simulink library "unity_lib_UDP"  (R2021a)
settings: Solver=VariableStepAuto  StartTime=0.0  StopTime=10.0  RelTol=1e-3
libraries: dspnetwork x1
settings Model: Creator=ge26jow  LastModifiedBy=ge26jow

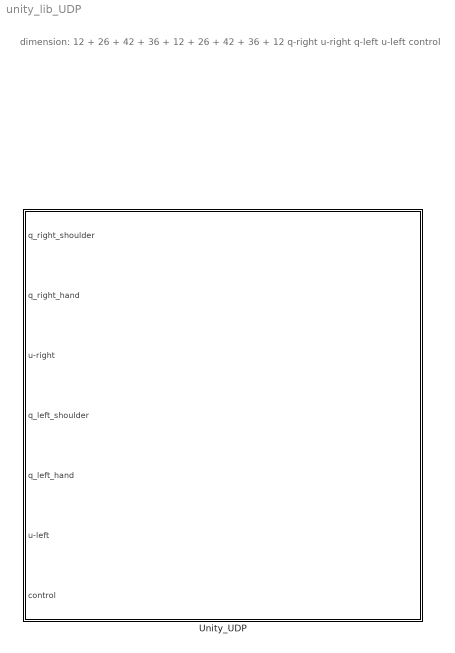
== system unity_lib_UDP ==
  note: dimension:
      |
      | 12 + 26 + 42 + 36 + 12 + 26 + 42 + 36 + 12
      | q-right u-right q-left u-left control
  Unity_UDP : Subsystem  mask{IP_port=8051, sampling_time=1e-2}
      mask prompts: IP_port "IP port"; sampling_time "sampling time"

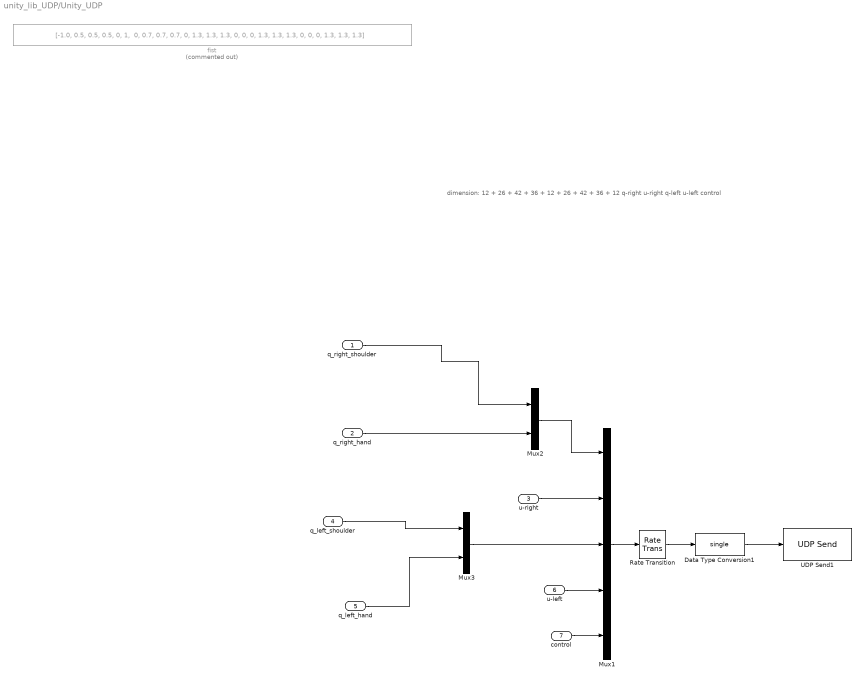
== system unity_lib_UDP/Unity_UDP ==
  note: dimension:
      |
      | 12 + 26 + 42 + 36 + 12 + 26 + 42 + 36 + 12
      | q-right u-right q-left u-left control
  q_right_shoulder : Inport
  q_right_hand : Inport  Port=2
  u-right : Inport  Port=3
  q_left_shoulder : Inport  Port=4
  q_left_hand : Inport  Port=5
  u-left : Inport  Port=6
  control : Inport  Port=7
  Data Type Conversion1 : DataTypeConversion  OutDataTypeStr=single
  Mux1 : Mux  Inputs=[12+26, 42+36, 12+26, 42+36, 12]
  Mux2 : Mux  Inputs=[12, 26]
  Mux3 : Mux  Inputs=[12, 26]
  Rate Transition : RateTransition  OutPortSampleTime=sampling_time
  UDP Send1 : dspnetwork/UDP Send  remoteURL='127.0.0.1'  remotePort=IP_port  localURL='0.0.0.0'  localPortSource=Automatically determine  localPort=-1  sendBufferSize=8192  sampletime=-1  blockPlatform=[]  separateLengthPort=0
      settings: SourceProductBaseCode=DS
  fist : Constant  Commented=on  Value="[-1.0, 0.5, 0.5, 0.5, 0, 1,  0, 0.7, 0.7, 0.7, 0, 1.3, 1.3, 1.3, 0, 0, 0, 1.3, 1.3, 1.3, 0, 0, 0, 1.3, 1.3, 1.3]"
  wires:
  q_right_hand/1 -> Mux2/2
  q_right_shoulder/1 -> Mux2/1
  Mux2/1 -> Mux1/1
  Mux3/1 -> Mux1/3
  Data Type Conversion1/1 -> UDP Send1/1
  Mux1/1 -> Rate Transition/1
  Rate Transition/1 -> Data Type Conversion1/1
  u-right/1 -> Mux1/2
  q_left_shoulder/1 -> Mux3/1
  q_left_hand/1 -> Mux3/2
  u-left/1 -> Mux1/4
  control/1 -> Mux1/5
